simulink model "AttitudeControlModel"  (R2018a)
settings: Solver=VariableStepAuto  StartTime=0.0  StopTime=10.0  RelTol=1e-3
undefined symbols (not defined in the file or in its folder): D, MOI
settings Model: Creator=Daniel  LastModifiedBy=Daniel

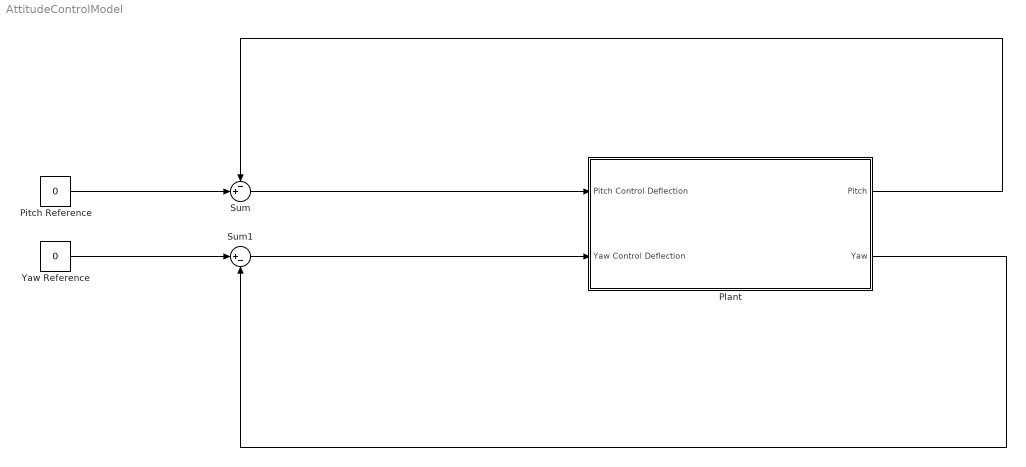
== system AttitudeControlModel ==
  Pitch Reference : Constant  Value=0
  Plant : Subsystem
  Sum : Sum  Inputs=-+|
  Sum1 : Sum  Inputs=|+-
  Yaw Reference : Constant  Value=0
  wires:
  Sum/1 -> Plant/1(Pitch Control Deflection)
  Pitch Reference/1 -> Sum/2
  Plant/1("Pitch ") -> Sum/1
  Yaw Reference/1 -> Sum1/1
  Sum1/1 -> Plant/2(Yaw Control Deflection)
  Plant/2(Yaw) -> Sum1/2

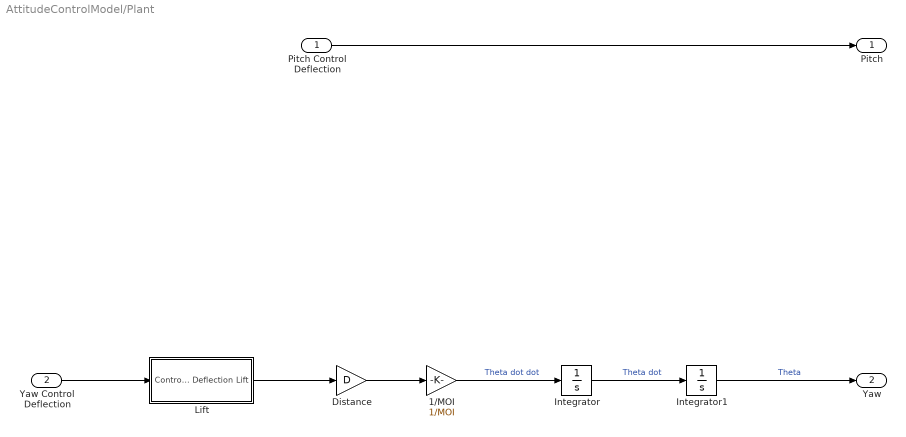
== system AttitudeControlModel/Plant ==
  Pitch Control Deflection : Inport
  Yaw Control Deflection : Inport  Port=2
  1/MOI : Gain  Gain=1/MOI
  Distance : Gain  Gain=D
  Integrator : Integrator
  Integrator1 : Integrator
  Lift : Subsystem
  "Pitch " : Outport
  Yaw : Outport  Port=2
  wires:
  Pitch Control Deflection/1 -> "Pitch "/1
  Integrator1/1 -> Yaw/1  "Theta"
  Integrator/1 -> Integrator1/1  "Theta dot"
  1/MOI/1 -> Integrator/1  "Theta dot dot"
  Yaw Control Deflection/1 -> Lift/1(Control Deflection)
  Lift/1(Lift) -> Distance/1
  Distance/1 -> 1/MOI/1

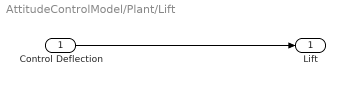
== system AttitudeControlModel/Plant/Lift ==
  Control Deflection : Inport
  Lift : Outport
  wires:
  Control Deflection/1 -> Lift/1
